simulink library "Gravity_Grad_Lib"  (R2018b)
settings: Solver=VariableStepAuto  StartTime=0.0  StopTime=10.0  RelTol=1e-3
settings Model: Creator=im11  LastModifiedBy=im11

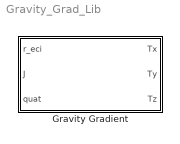
== system Gravity_Grad_Lib ==
  Gravity Gradient : Subsystem

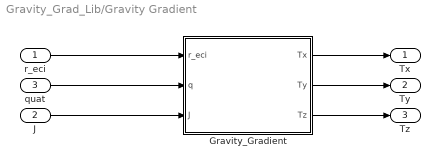
== system Gravity_Grad_Lib/Gravity Gradient ==
  r_eci : Inport
  J : Inport  Port=2
  quat : Inport  Port=3
  "Gravity_Gradient " : MATLAB Function  TreatAsAtomicUnit=on
  Tx : Outport
  Ty : Outport  Port=2
  Tz : Outport  Port=3
  wires:
  "Gravity_Gradient "/1(Tx) -> Tx/1
  "Gravity_Gradient "/2(Ty) -> Ty/1
  "Gravity_Gradient "/3(Tz) -> Tz/1
  r_eci/1 -> "Gravity_Gradient "/1(r_eci)
  quat/1 -> "Gravity_Gradient "/2(q)
  J/1 -> "Gravity_Gradient "/3(J)

== matlab function Gravity_Grad_Lib/Gravity Gradient/Gravity_Gradient  ==
  data: r_eci input; Tx output; q input; Ty output; Tz output; J input
function [Tx,Ty,Tz] = fcn(r_eci,q,J)
%r_eci is the position vector in the reci coord frame in meters
%J is the moment of inertia
%q is the unit quaternion 
%This will output the gravity gradients from the position 


RAD2DEG = 180/pi;
DEG2RAD = pi/180;

r_eci = r_eci/1000; %converting to meters
EUL = quat2eul(q);

mu = 3.986004418e14; % in m^3/s^2
Ro = sqrt(r_eci(1)^2+r_eci(2)^2+r_eci(3)^2);


Tx = 3*mu/(2*Ro^3)*(J(3)-J(2))sin(2*Eul(2))*cos(Eul(1))^2;
Ty = 3*mu/(2*Ro^3)*(J(3)-J(1))sin(2*Eul(1))*cos(Eul(2))^2;
Tz = 3*mu/(2*Ro^3)*(J(1)-J(2))sin(2*Eul(1))*cos(Eul(2))^2;


end
